simulink model "First_second_order"  (R2023a)
settings: Solver=ode23t  StartTime=0.0  StopTime=2000  FixedStep=1e-2  MaxStep=0.01  RelTol=1e-3  EnableMultiTasking=on
InitFcn:
  | load('VOC_1C_3pulse_14rest.mat')
  | 
  | %Rp1 = 0.0146;
  | %Rp2 = 0.0084;
  | %Cp1 = 2.1967e+03;
  | %Cp2 = 2.1298e+04;
  | 
  | Rp1 = 0.0099;
  | Rp2 = 0.0375;
  | Cp1 = 1.1826e+03;
  | Cp2 = 3.1373e+03;
undefined symbols (not defined in the file): Cp, Rp, Rs, SOC, voc_sort
libraries: simulink x2
settings Model: Creator=Volan  LastModifiedBy=gabrielcrisan
settings SolverCC: AlgebraicLoopSolver=LineSearch
settings DataIOCC: LimitDataPoints=on  SaveFormat=Array  ReturnWorkspaceOutputs=off
settings OptimizationCC: LifeSpan=inf
settings DebuggingCC: UnderspecifiedInitializationDetection=Classic  MergeDetectMultiDrivingBlocksExec=none  SolverPrmCheckMsg=warning  UnconnectedInputMsg=warning  UnconnectedOutputMsg=warning  UnconnectedLineMsg=warning  SFUnexpectedBacktrackingDiag=warning  SFNoUnconditionalDefaultTransitionDiag=warning  SFExecutionAtInitializationDiag=none  ArithmeticOperatorsInVariantConditions=warning
settings HardwareCC: ProdBitPerPointer=32  ProdBitPerSizeT=32  ProdBitPerPtrDiffT=32  ProdLargestAtomicFloat=None  ProdIntDivRoundTo=Undefined  ProdEndianess=Unspecified  ProdWordSize=32  ProdHWDeviceType=32-bit Generic
settings ModelReferenceCC: EnableRefExpFcnMdlSchedulingChecks=on  PropagateSignalLabelsOutOfModel=off
settings SFSimCC: SimUseLocalCustomCode=off  CustomCodeUndefinedFunction=UseInterfaceOnly
settings RTWCC: RTWUseLocalCustomCode=off
settings CodeAppCC: StateflowObjectComments=on
settings GRTTargetCC: TargetLangStandard=C89/C90 (ANSI)
settings ConfigComp: CovMetricSettings=dw  CovSaveCumulativeToWorkspaceVar=on  CovSaveSingleToWorkspaceVar=on  CovExternalEMLEnable=off
settings SimscapeCC: SimscapeNormalizeSystem=off
settings ConfigurationSet: Description=SimMechanics 2G

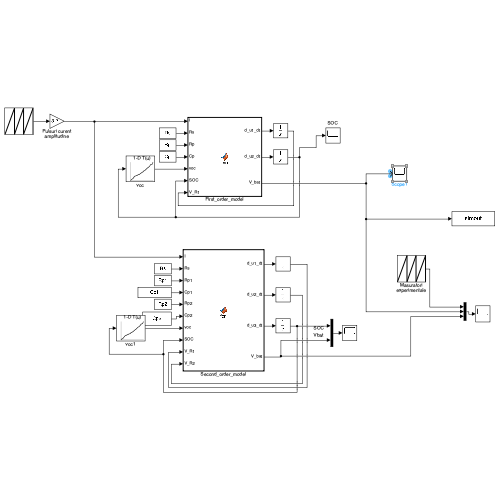
[thumbnail: Simulink's stored preview of the top-level diagram]
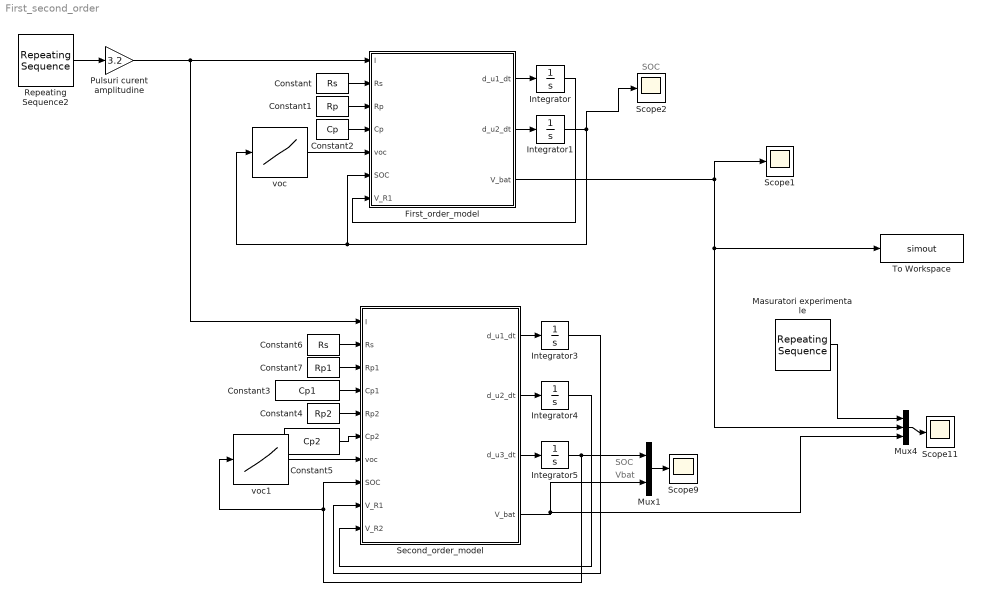
== system First_second_order ==
  note: SOC
  note: Vbat
  note: SOC
  Constant : Constant  Value=Rs
  Constant1 : Constant  Value=Rp
  Constant2 : Constant  Value=Cp
  Constant3 : Constant  Value=Cp1
  Constant4 : Constant  Value=Rp2
  Constant5 : Constant  Value=Cp2
  Constant6 : Constant  Value=Rs
  Constant7 : Constant  Value=Rp1
  First_order_model : MATLAB Function  TreatAsAtomicUnit=on
  Integrator : Integrator
  Integrator1 : Integrator  InitialCondition=100
  Integrator3 : Integrator
  Integrator4 : Integrator
  Integrator5 : Integrator  InitialCondition=100
  Masuratori experimentale : simulink/Sources/Repeating Sequence  rep_seq_t=time  rep_seq_y=Vbat
  Mux1 : Mux  Inputs=2
  Mux4 : Mux  Inputs=3
  Pulsuri curent amplitudine : Gain  Gain=3.2
  Repeating Sequence2 : simulink/Sources/Repeating Sequence  rep_seq_t=time  rep_seq_y=pulse
  Scope{1..2,9,11} (4 alike) : Scope
  Second_order_model : MATLAB Function  TreatAsAtomicUnit=on
  To Workspace : ToWorkspace  VariableName=simout  SaveFormat=Timeseries  SampleTime=-1
  voc : Lookup_n-D  NumberOfTableDimensions=1  BreakpointsForDimension1=SOC  Table=voc_sort  InternalRulePriority=Speed  RndMeth=Simplest
  voc1 : Lookup_n-D  NumberOfTableDimensions=1  BreakpointsForDimension1=SOC  Table=voc_sort  InternalRulePriority=Speed  RndMeth=Simplest
  wires:
  voc/1 -> First_order_model/5(voc)
  First_order_model/1(d_u1_dt) -> Integrator/1
  Integrator/1 -> First_order_model/7(V_R1)
  First_order_model/2(d_u2_dt) -> Integrator1/1
  Integrator1/1 -> voc/1, First_order_model/6(SOC), Scope2/1
  Constant/1 -> First_order_model/2(Rs)
  Constant1/1 -> First_order_model/3(Rp)
  Constant2/1 -> First_order_model/4(Cp)
  Repeating Sequence2/1 -> Pulsuri curent amplitudine/1
  Second_order_model/1(d_u1_dt) -> Integrator3/1
  Constant6/1 -> Second_order_model/2(Rs)
  Second_order_model/2(d_u2_dt) -> Integrator4/1
  voc1/1 -> Second_order_model/7(voc)
  Constant4/1 -> Second_order_model/5(Rp2)
  Integrator5/1 -> voc1/1, Second_order_model/8(SOC), Mux1/1
  Second_order_model/4(V_bat) -> Mux4/3, Mux1/2
  Constant3/1 -> Second_order_model/4(Cp1)
  Masuratori experimentale/1 -> Mux4/1
  Constant7/1 -> Second_order_model/3(Rp1)
  Integrator4/1 -> Second_order_model/10(V_R2)
  Constant5/1 -> Second_order_model/6(Cp2)
  Integrator3/1 -> Second_order_model/9(V_R1)
  Pulsuri curent amplitudine/1 -> Second_order_model/1(I), First_order_model/1(I)
  Second_order_model/3(d_u3_dt) -> Integrator5/1
  Mux1/1 -> Scope9/1
  Mux4/1 -> Scope11/1
  First_order_model/3(V_bat) -> To Workspace/1, Mux4/2, Scope1/1

== matlab function First_second_order/Second_order_model ==
  data: I input; Rs input; Rp1 input; Cp1 input; Rp2 input; Cp2 input; voc input; d_u1_dt output; SOC input; V_R1 input; V_R2 input; d_u2_dt output; d_u3_dt output; V_bat output
function [d_u1_dt,d_u2_dt,d_u3_dt,V_bat] = fcn(I,Rs,Rp1,Cp1,Rp2,Cp2,voc,SOC,V_R1,V_R2)


Q = 3.2*3600/1e2; %[Ah]

%States
u1 = V_R1;
u2 = V_R2;
u3 = SOC;

d_u1_dt = (-1/(Rp1*Cp1))*u1 - (I/Cp1);
d_u2_dt = (-1/(Rp2*Cp2))*u2 - (I/Cp2);
d_u3_dt = -I/Q;

V_bat = voc + u1 + u2 - Rs*I;

== matlab function First_second_order/First_order_model ==
  data: I input; Rs input; Rp input; Cp input; voc input; d_u1_dt output; SOC input; V_R1 input; d_u2_dt output; V_bat output
function [d_u1_dt,d_u2_dt,V_bat] = fcn(I,Rs,Rp,Cp,voc,SOC,V_R1)


Q = 3.2*3600/1e2; %[Ah]


%States
u1 = V_R1;
u2 = SOC;

d_u1_dt = -1/(Rp*Cp)*u1 + (1/Cp)*I;

d_u2_dt = -I/Q;

V_bat = voc - u1 - Rs*I;
